simulink model "PQRECTer"  (R2020b)
settings: Solver=VariableStepAuto  StartTime=0.0  StopTime=0.5  RelTol=1e-3
libraries: powerlib x10, powerlib_meascontrol x3, simulink x2, pid_lib x1, powerlib_extras x1
settings Model: SimulationMode=accelerator  Creator=岉  LastModifiedBy=86130

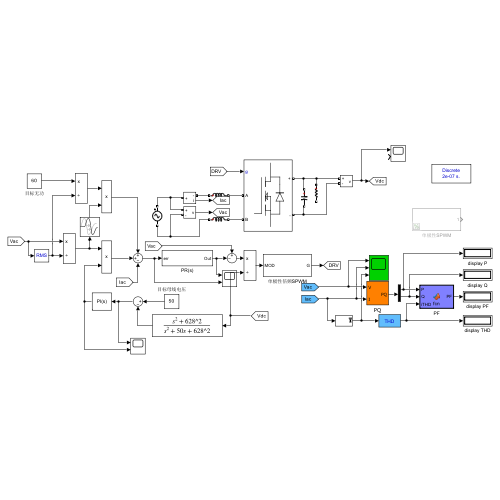
[thumbnail: Simulink's stored preview of the top-level diagram]
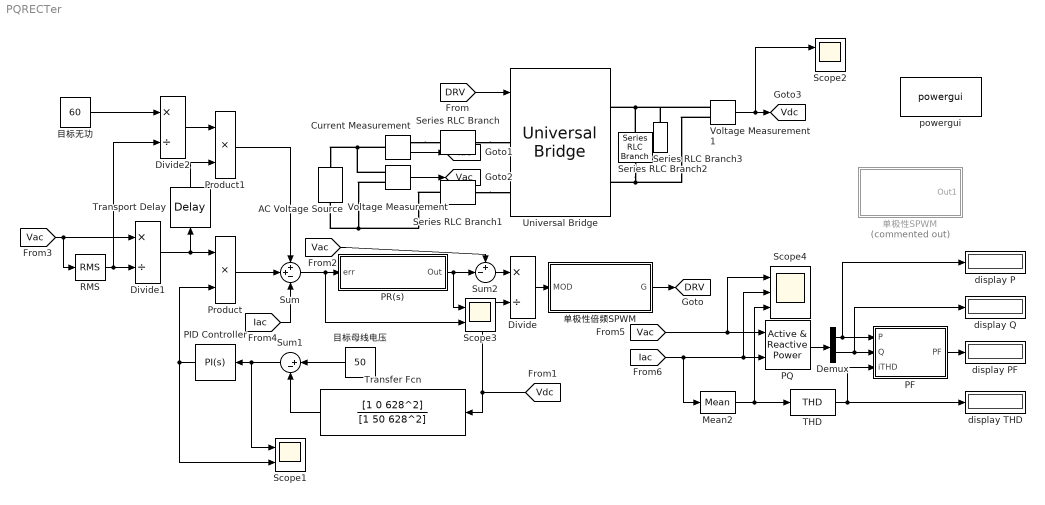
== system PQRECTer ==
  AC Voltage Source : powerlib/Electrical Sources/AC Voltage Source  Amplitude=30*1.41  Phase=0  Frequency=50  SampleTime=0  Measurements=None  BusType=swing  Pref=10e3  Qref=0  Qmin=-inf  Qmax=+inf
  Current Measurement : powerlib/Measurements/Current Measurement  PhasorSimulation=off  OutputType=Complex  PSBequivalent=0
  Demux : Demux  Outputs=2
  Divide : Product  Inputs=*/
  Divide1 : Product  Inputs=*/
  Divide2 : Product  Inputs=*/
  Mean2 : powerlib_meascontrol/Measurements/Mean  Freq=20000  Vinit=0  Ts=0
  PF : MATLAB Function  TreatAsAtomicUnit=on
  PID Controller : pid_lib/PID Controller  Controller=PI  Form=Parallel  TimeDomain=Continuous-time  UseExternalTs=off  SampleTime=-1  IntegratorMethod=Forward Euler  ControllerParametersSource=internal  P=0.15  I=6  D=0  N=100  UseFilter=on  TunerSelectOption=Transfer Function Based (PID Tuner App)  InitialConditionSource=internal  InitialConditionForIntegrator=0  InitialConditionForFilter=0  DifferentiatorICPrevScaledInput=0  ExternalReset=none  TrackingMode=off  Kt=1  LimitOutput=off  SatLimitsSource=internal  UpperSaturationLimit=inf  LowerSaturationLimit=-inf  LinearizeAsGain=on  AntiWindupMode=none  Kb=1  POutMin=[]  POutMax=[]  IOutMin=[]  IOutMax=[]  DOutMin=[]  DOutMax=[]  NOutMin=[]  NOutMax=[]  SumOutMin=[]  SumOutMax=[]  SaturationOutMin=[]  SaturationOutMax=[]  PParamMin=[]  PParamMax=[]  IParamMin=[]  IParamMax=[]  DParamMin=[]  DParamMax=[]  NParamMin=[]  NParamMax=[]  KbParamMin=[]  KbParamMax=[]  KtParamMin=[]  KtParamMax=[]  KbOutMin=[]  KbOutMax=[]  KtOutMin=[]  KtOutMax=[]  IntegratorOutMin=[]  IntegratorOutMax=[]  FilterOutMin=[]  FilterOutMax=[]  SumI1OutMin=[]  SumI1OutMax=[]  SumI2OutMin=[]  SumI2OutMax=[]  SumI3OutMin=[]  SumI3OutMax=[]  SumI4OutMin=[]  SumI4OutMax=[]  SumDOutMin=[]  SumDOutMax=[]  DifferentiatorOutMin=[]  DifferentiatorOutMax=[]  FilterDiffOutCoefMin=[]  FilterDiffOutCoefMax=[]  ReciprocalOutMin=[]  ReciprocalOutMax=[]  SumDenOutMin=[]  SumDenOutMax=[]  SumNumOutMin=[]  SumNumOutMax=[]  DivideOutMin=[]  DivideOutMax=[]  UdiffTsProdOutMin=[]  UdiffTsProdOutMax=[]  NTsProdOutMin=[]  NTsProdOutMax=[]  UintegralTsProdOutMin=[]  UintegralTsProdOutMax=[]  UngainTsProdOutMin=[]  UngainTsProdOutMax=[]  IntegratorContinuousStateAttributes=''  IntegratorStateMustResolveToSignalObject=off  IntegratorRTWStateStorageClass=Auto  FilterContinuousStateAttributes=''  FilterStateMustResolveToSignalObject=off  FilterRTWStateStorageClass=Auto  ParallelPVariant=InternalParameters  IdealPVariant=Disabled  IVariant=InternalParameters  DVariant=Disabled  IntegratorVariant=Continuous  SatVariant=Disabled  AWVariant=Passthrough  PCopyVariant=Disabled  TRVariant=Disabled  FdbkBlocksVariant=Forward  IdealPFdbkVariant=Disabled  SatFdbkVariant=Disabled  DerivativeFilterVariant=Disabled  NVariant=Disabled  NCopyVariant=Disabled_SignalSpec  FilterICVariant=Disabled  IntegratorICVariant=InternalICs  ExternalResetVariant=Disabled  TRSumVariant=Passthrough  SumFdbkVariant=Disabled  SumVariant=Sum_PI  TsampFilterVariant=InternalTs  TsampNgainVariant=Passthrough  TsampIntegralVariant=Disabled_SignalSpec  ExternalSaturationOutDataTypeStr=Inherit: Same as second input
  PQ : powerlib_extras/Measurements/Active & Reactive Power  f1=50
  PR(s) : Subsystem
  Product : Product
  Product1 : Product
  RMS : powerlib_meascontrol/Measurements/RMS  TrueRMS=off  Freq=50  RMSInit=30  Ts=0
  Scope1 : Scope  NumInputPorts=2
  Scope2 : Scope  NumInputPorts=2
  Scope3 : Scope  NumInputPorts=2
  Scope4 : Scope  NumInputPorts=3
  Series RLC Branch : powerlib/Elements/Series RLC Branch  LConnTagsString=__new0  RConnTagsString=__new0  BranchType=L  Resistance=1  Inductance=4.7e-4  SetiL0=off  InitialCurrent=0  Capacitance=1e-6  Setx0=off  InitialVoltage=0  Measurements=None
  Series RLC Branch1 : powerlib/Elements/Series RLC Branch  LConnTagsString=__new0  RConnTagsString=__new0  BranchType=L  Resistance=1  Inductance=4.7e-4  SetiL0=off  InitialCurrent=0  Capacitance=1e-6  Setx0=off  InitialVoltage=0  Measurements=None
  Series RLC Branch2 : powerlib/Elements/Series RLC Branch  LConnTagsString=__new0  RConnTagsString=__new0  BranchType=C  Resistance=1  Inductance=4.7e-4  SetiL0=off  InitialCurrent=0  Capacitance=2e-3  Setx0=on  InitialVoltage=42  Measurements=None
  Series RLC Branch3 : powerlib/Elements/Series RLC Branch  LConnTagsString=__new0  RConnTagsString=__new0  BranchType=R  Resistance=40  Inductance=4.7e-4  SetiL0=off  InitialCurrent=0  Capacitance=1e-6  Setx0=off  InitialVoltage=0  Measurements=None
  Sum : Sum  Inputs=++-
  Sum1 : Sum  Inputs=|+-
  Sum2 : Sum  Inputs=+-|
  THD : powerlib_meascontrol/Measurements/THD  Freq=50  Ts=0
  Transfer Fcn : TransferFcn  Numerator=[1 0 628^2]  Denominator=[1 50 628^2]
  Transport Delay : TransportDelay  DelayTime=0.005
  Universal Bridge : powerlib/Power Electronics/Universal Bridge  Arms=2  SnubberResistance=1e5  SnubberCapacitance=inf  Device=MOSFET / Diodes  Ron=1e-2  Lon=0  ForwardVoltages="[  0  0  ]"  ForwardVoltage=0  GTOparameters=[ 10e-6 , 20e-6 ]  IGBTparameters=[ 1e-6 , 2e-6 ]  Measurements=None  Measurements_2=None  converterType=Rectifier
  Voltage Measurement : powerlib/Measurements/Voltage Measurement  PhasorSimulation=off  OutputType=Complex  PSBequivalent=0
  Voltage Measurement1 : powerlib/Measurements/Voltage Measurement  PhasorSimulation=off  OutputType=Complex  PSBequivalent=0
  display P : Display
  display PF : Display
  display Q : Display
  display THD : Display
  powergui : powerlib/powergui  Priority=1  SimulationMode=Discrete  SampleTime=2e-7  frequency=60  Iterations=50  frequencyindice=0  Pbase=100e6  ErrMax=1e-4  UnitsV=kV  UnitsW=MW  buscounter=0  FunctionMessages=off  echomessages=off  EnableUseOfTLC=off  CurrentSourceSwitches=off  DisableSnubberDevices=off  DisableRonSwitches=off  DisableVfSwitches=off  DisplayEquations=off  AutomaticDiscreteSolvers=off  SolverType=Tustin/Backward Euler (TBE)  Interpol=off  ExternalGateDelay=off  methode=off  Ts=100  x0status=blocks  SPID=on  SwTol=0  HookPort=off  NonlinearTolerance=1e-4  nMaxIteration=100  ContinueOnMaxIteration=off  RestoreLinks=warning  ResistiveCurrentMeasurement=off  Frange=[0:2:500]  Ylog=off  Xlog=on  ShowGrid=off  save=off  variable=ZData  structure=0  ZoomFFT=off  StartTime=0.0  cycles=1  DisplayStyle=1  fundamental=60  FreqAxis=off  MaxFrequency=1000  frequencyindicesteady=1  RmsSteady=1  display=off
  单极性SPWM : Subsystem  Commented=on
  单极性倍频SPWM : Subsystem
  目标无功 : Constant  Value=60
  目标母线电压 : Constant  Value=50
  tag scope: DRV=global, Iac=global, Vac=global, Vdc=global
  wires:
  单极性倍频SPWM/1(G) -> [DRV]
  [DRV] -> Universal Bridge/1
  Current Measurement/1 -> [Iac]
  Voltage Measurement/1 -> [Vac]
  THD/1 -> display THD/1, PF/3(iTHD)
  [Iac] -> Mean2/1, Scope4/2, PQ/2
  PF/1(PF) -> display PF/1
  Mean2/1 -> Scope4/3, THD/1
  PQ/1 -> Demux/1
  Demux/1 -> display P/1, PF/1(P)
  [Vac] -> Scope4/1, PQ/1
  Demux/2 -> display Q/1, PF/2(Q)
  Voltage Measurement1/1 -> Scope2/1, [Vdc]
  目标母线电压/1 -> Sum1/1
  [Vdc] -> Transfer Fcn/1, Divide/2
  Sum1/1 -> Scope1/1, PID Controller/1
  PID Controller/1 -> Scope1/2, Product/2
  PR(s)/1(Out) -> Scope3/1, Sum2/2
  [Vac] -> Sum2/1
  Divide/1 -> 单极性倍频SPWM/1(MOD)
  Sum2/1 -> Divide/1
  Sum/1 -> Scope3/2, PR(s)/1(err)
  Transfer Fcn/1 -> Sum1/2
  Divide1/1 -> Product/1, Transport Delay/1
  [Iac] -> Sum/3
  Product/1 -> Sum/2
  Transport Delay/1 -> Product1/2
  Product1/1 -> Sum/1
  [Vac] -> Divide1/1, RMS/1
  RMS/1 -> Divide1/2, Divide2/2
  Divide2/1 -> Product1/1
  目标无功/1 -> Divide2/1
  connections:
  Series RLC Branch/RConn1 -- Universal Bridge/LConn1
  Series RLC Branch1/RConn1 -- Universal Bridge/LConn2
  Current Measurement/RConn1 -- Series RLC Branch/LConn1
  Current Measurement/LConn1 -- Voltage Measurement/LConn1 -- AC Voltage Source/RConn1
  Series RLC Branch1/LConn1 -- AC Voltage Source/LConn1 -- Voltage Measurement/LConn2
  Series RLC Branch2/LConn1 -- Series RLC Branch3/LConn1 -- Voltage Measurement1/LConn1 -- Universal Bridge/RConn1
  Series RLC Branch2/RConn1 -- Voltage Measurement1/LConn2 -- Universal Bridge/RConn2

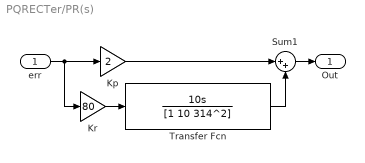
== system PQRECTer/PR(s) ==
  err : Inport
  Kp : Gain  Gain=2
  Kr : Gain  Gain=80
  Sum1 : Sum  Inputs=|++
  Transfer Fcn : TransferFcn  Numerator=[10 0]  Denominator=[1 10 314^2]
  Out : Outport
  wires:
  Kp/1 -> Sum1/1
  Transfer Fcn/1 -> Sum1/2
  err/1 -> Kr/1, Kp/1
  Kr/1 -> Transfer Fcn/1
  Sum1/1 -> Out/1

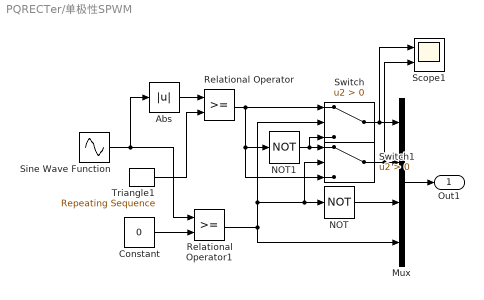
== system PQRECTer/单极性SPWM ==
  Abs : Abs
  Constant : Constant  Value=0
  Mux : Mux
  NOT : Logic  Operator=NOT  IconShape=distinctive  AllPortsSameDT=off  OutDataTypeStr=boolean
  NOT1 : Logic  Operator=NOT  IconShape=distinctive  AllPortsSameDT=off  OutDataTypeStr=boolean
  Relational Operator : RelationalOperator  OutDataTypeStr=boolean  RndMeth=Simplest
  Relational Operator1 : RelationalOperator  OutDataTypeStr=boolean  RndMeth=Simplest
  Scope1 : Scope  NumInputPorts=2
  Sine Wave Function : Sin  Frequency=314  SampleTime=0
  Switch : Switch  Criteria=u2 > Threshold
  Switch1 : Switch  Criteria=u2 > Threshold
  Triangle1 : simulink/Sources/Repeating Sequence  rep_seq_t=[0 1/20000/2 1/20000]  rep_seq_y=[0 1 0]
  Out1 : Outport
  wires:
  Mux/1 -> Out1/1
  Triangle1/1 -> Relational Operator/2
  Constant/1 -> Relational Operator1/2
  NOT/1 -> Mux/3
  Relational Operator1/1 -> Mux/4, Switch1/2, NOT/1, Switch/2
  Switch/1 -> Scope1/1, Mux/1
  Switch1/1 -> Scope1/2, Mux/2
  Relational Operator/1 -> Switch1/3, NOT1/1, Switch/1
  NOT1/1 -> Switch1/1, Switch/3
  Abs/1 -> Relational Operator/1
  Sine Wave Function/1 -> Abs/1, Relational Operator1/1

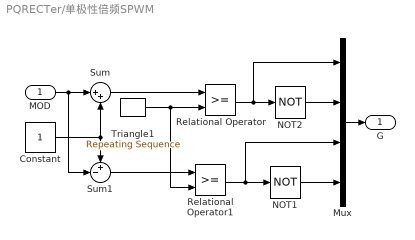
== system PQRECTer/单极性倍频SPWM ==
  MOD : Inport
  Constant : Constant
  Mux : Mux
  NOT1 : Logic  Operator=NOT  IconShape=distinctive  AllPortsSameDT=off  OutDataTypeStr=boolean
  NOT2 : Logic  Operator=NOT  IconShape=distinctive  AllPortsSameDT=off  OutDataTypeStr=boolean
  Relational Operator : RelationalOperator  OutDataTypeStr=boolean  RndMeth=Simplest
  Relational Operator1 : RelationalOperator  OutDataTypeStr=boolean  RndMeth=Simplest
  Sum : Sum  Inputs=|++
  Sum1 : Sum  Inputs=+-|
  Triangle1 : simulink/Sources/Repeating Sequence  rep_seq_t=[0 1/20000/2 1/20000]  rep_seq_y=[0 2 0]
  G : Outport
  wires:
  MOD/1 -> Sum1/2, Sum/1
  Mux/1 -> G/1
  Constant/1 -> Sum/2, Sum1/1
  Sum/1 -> Relational Operator/1
  Triangle1/1 -> Relational Operator1/2, Relational Operator/2
  Relational Operator/1 -> NOT2/1, Mux/1
  Sum1/1 -> Relational Operator1/1
  Relational Operator1/1 -> Mux/3, NOT1/1
  NOT1/1 -> Mux/4
  NOT2/1 -> Mux/2

== matlab function PQRECTer/PF ==
  data: P input; PF output; Q input; iTHD input
function PF = fcn(P,Q,iTHD)
% This block supports an embeddable subset of the MATLAB language.
% See the help menu for details. 
PF=(P/sqrt(P*P+Q*Q))/(sqrt(1+iTHD*iTHD));
